simulink model "read_agg_ctrl_simulated_loads_example"  (R2015a)
settings: Solver=ode45  SolverMode=SingleTasking  StartTime=0.0  StopTime=10.0  RelTol=1e-3
libraries: libAggregators x1, libSimulators x1, libControllers x1
settings Model: Creator=jcardena  LastModifiedBy=BCao
settings OptimizationCC: BlockReduction=off  BooleanDataType=off
settings DebuggingCC: SaveWithParameterizedLinksMsg=none  UnderspecifiedInitializationDetection=Classic  MergeDetectMultiDrivingBlocksExec=none  SignalResolutionControl=TryResolveAllWithWarning  StrictBusMsg=Warning
settings HardwareCC: TargetUnknown=on

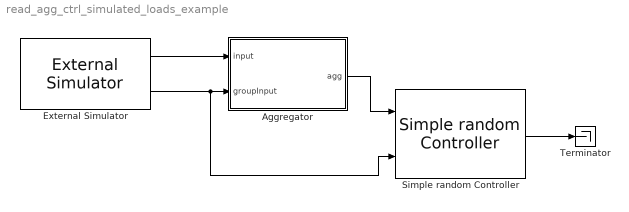
== system read_agg_ctrl_simulated_loads_example ==
  Aggregator : Subsystem  BlockChoice=Simplest
      settings: AttributesFormatString=%<BlockChoice>  TemplateBlock=libAggregators/Aggregator  MemberBlocks=Average,Simple,Simple db Aggregator,Simplest
  External Simulator : libSimulators/External Simulator  Condition=%20151213%  N=10  db_name=HeatingUnits  db_username=sw_ETS  db_password=unb.sql.2015
  Simple random Controller : libControllers/Simple random Controller  db_name=HeatingUnits  db_username=sw_ETS  db_password=unb.sql.2015
  Terminator : Terminator
  wires:
  External Simulator/2 -> Simple random Controller/2, Aggregator/2(groupInput)
  External Simulator/1 -> Aggregator/1(input)
  Aggregator/1(agg) -> Simple random Controller/1
  Simple random Controller/1 -> Terminator/1

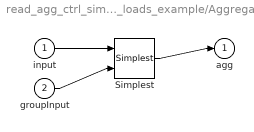
== system read_agg_ctrl_simulated_loads_example/Aggregator ==
  input : Inport
  groupInput : Inport  Port=2
  Simplest : libAggregators/Simplest  SystemSampleTime=-1
  agg : Outport
  wires:
  input/1 -> Simplest/1
  groupInput/1 -> Simplest/2
  Simplest/1 -> agg/1
